simulink model "Motormodel"  (R2014b)
settings: Solver=ode23t  StartTime=0.0  StopTime=10.0  RelTol=1e-3
values from neighbouring files (symbols this model uses):
  J = 138E-7    (= 1.38e-05)    [gs.m]
  K_emf = 1/158    (= 0.00632911392405)    [gs.m]
  Kt = 60.3E-3    (= 0.0603)    [gs.m]
  L = 0.329E-3    (= 0.000329)    [gs.m]
  max_current = 4    [gs.m]
  Rm = 1.16    [gs.m]
  X0 = x0    [gs.m]
settings Model: Creator=MikaelSjostedt  LastModifiedBy=MikaelSjostedt

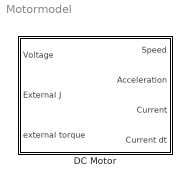
== system Motormodel ==
  DC Motor : Subsystem

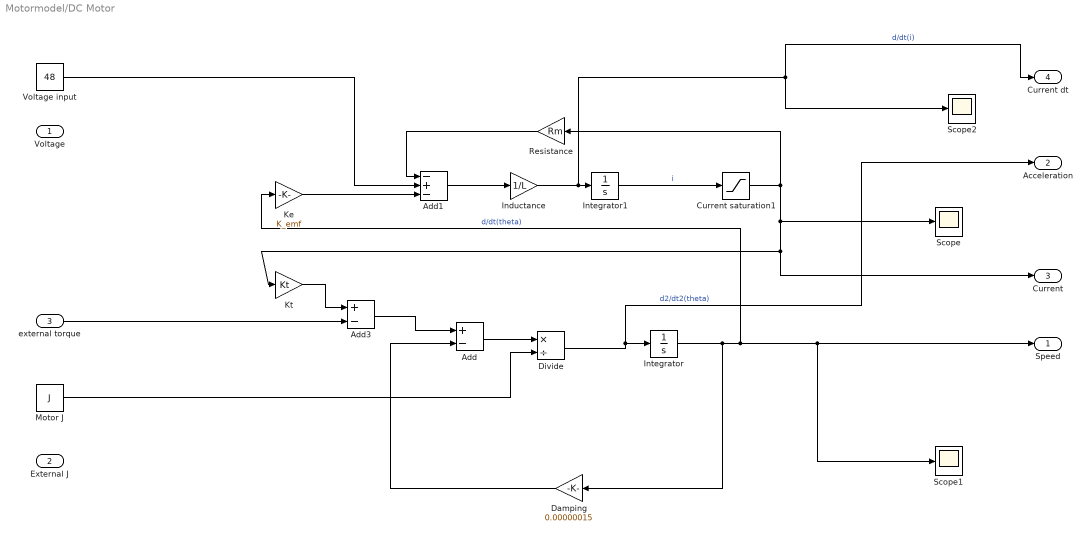
== system Motormodel/DC Motor ==
  Voltage : Inport
  External J : Inport  Port=2
  "external torque " : Inport  Port=3
  Add : Sum  Inputs=+-
  Add1 : Sum  Inputs=-+-
  Add3 : Sum  Inputs=+-
  Current saturation1 : Saturate  UpperLimit=max_current  LowerLimit=-max_current
  Damping : Gain  Gain=0.00000015
  Divide : Product  Inputs=*/
  Inductance : Gain  Gain=1/L
  Integrator : Integrator  InitialCondition=X0(2)
  Integrator1 : Integrator
  Ke : Gain  Gain=K_emf
  Kt : Gain  Gain=Kt
  "Motor J " : Constant  Value=J
  Resistance : Gain  Gain=Rm
  Scope : Scope
      settings: SaveName=ScopeData7
  Scope1 : Scope
      settings: SaveName=ScopeData8
  Scope2 : Scope
      settings: SaveName=ScopeData9
  "Voltage input " : Constant  Value=48
  " Speed" : Outport
  Acceleration : Outport  Port=2
  Current : Outport  Port=3
  Current dt : Outport  Port=4
  wires:
  Integrator1/1 -> Current saturation1/1  "i"
  Inductance/1 -> Integrator1/1, Scope2/1, Current dt/1  "d/dt(i)"
  Divide/1 -> Acceleration/1, Integrator/1  "d2/dt2(theta)"
  Integrator/1 -> Ke/1, Scope1/1, " Speed"/1, Damping/1  "d/dt(theta)"
  Add1/1 -> Inductance/1
  Add/1 -> Divide/1
  Damping/1 -> Add/2
  Kt/1 -> Add3/1
  Resistance/1 -> Add1/1
  Ke/1 -> Add1/3
  "Motor J "/1 -> Divide/2
  Add3/1 -> Add/1
  "external torque "/1 -> Add3/2
  Current saturation1/1 -> Scope/1, Current/1, Kt/1, Resistance/1
  "Voltage input "/1 -> Add1/2
